simulink model "pidDesigne"  (R2018a)
settings: Solver=VariableStepAuto  StartTime=0.0  StopTime=10.0  RelTol=1e-3
settings Model: Creator=misar  LastModifiedBy=misar

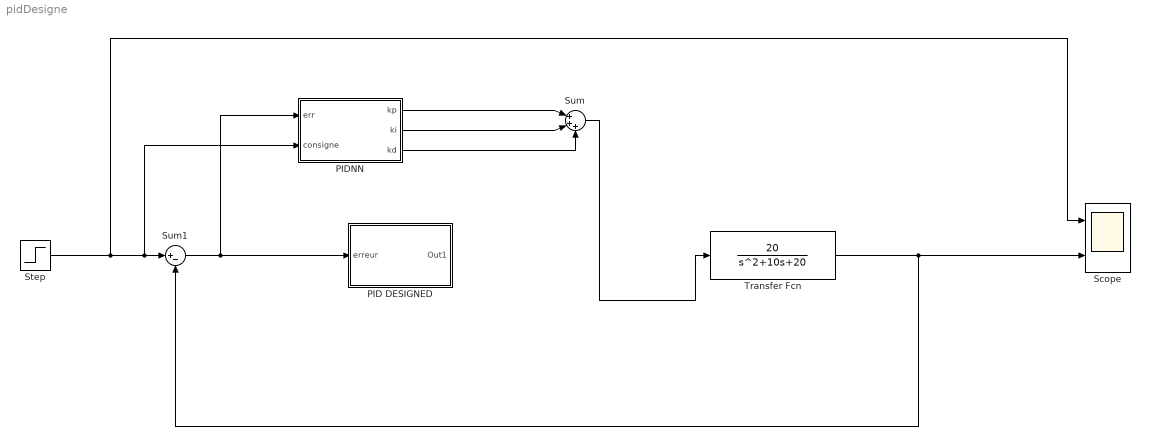
== system pidDesigne ==
  "PID DESIGNED " : Subsystem
  PIDNN : Subsystem
  Scope : Scope  NumInputPorts=2
  Step : Step  Time=0  SampleTime=0
  Sum : Sum  Inputs=|+++
  Sum1 : Sum  Inputs=|+-
  Transfer Fcn : TransferFcn  Numerator=[20]  Denominator=[1 10 20]
  wires:
  Transfer Fcn/1 -> Scope/2, Sum1/2
  Step/1 -> PIDNN/2("consigne "), Sum1/1, Scope/1
  Sum1/1 -> "PID DESIGNED "/1(erreur), PIDNN/1("err ")
  PIDNN/1(kp) -> Sum/1
  PIDNN/2(ki) -> Sum/2
  PIDNN/3(kd) -> Sum/3
  Sum/1 -> Transfer Fcn/1

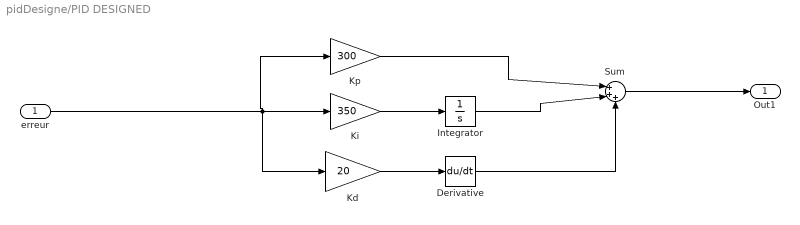
== system pidDesigne/PID DESIGNED  ==
  erreur : Inport
  Derivative : Derivative
  Integrator : Integrator
  Kd : Gain  Gain=20
  Ki : Gain  Gain=350
  Kp : Gain  Gain=300
  Sum : Sum  Inputs=|+++
  Out1 : Outport
  wires:
  Integrator/1 -> Sum/2
  Derivative/1 -> Sum/3
  Kp/1 -> Sum/1
  Kd/1 -> Derivative/1
  Ki/1 -> Integrator/1
  Sum/1 -> Out1/1
  erreur/1 -> Kd/1, Kp/1, Ki/1

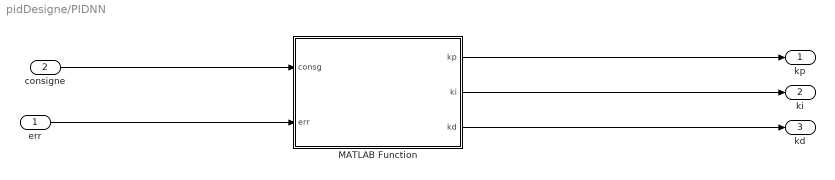
== system pidDesigne/PIDNN ==
  "err " : Inport
  "consigne " : Inport  Port=2
  MATLAB Function : MATLAB Function  TreatAsAtomicUnit=on
  kp : Outport
  ki : Outport  Port=2
  kd : Outport  Port=3
  wires:
  MATLAB Function/2(ki) -> ki/1
  MATLAB Function/3(kd) -> kd/1
  MATLAB Function/1(kp) -> kp/1
  "err "/1 -> MATLAB Function/2(err)
  "consigne "/1 -> MATLAB Function/1(consg)

== matlab function pidDesigne/PIDNN/MATLAB Function ==
  data: consg input; err input; kp output; ki output; kd output
function [kp,ki,kd]=  err(consg, err)
    epochs = 150000;
    learningRate = 0.01;
    w1=1;
    w2=1;
    w3=1;
    for i=0:epochs
        [a1 , kp ,a2,ki,a3,kd] = forward(err,w1,w2,w3);
        [theata2,theata3,theata4 ]= backProbagation(w2,a2,err,z1,z2,y);
        w1= w1-learningRate*(1/lenght(err))*theata3;
        w1= w2-learningRate*(1/lenght(err))*theata1;
        
    end 



end
